simulink model "RampModelRunner"  (R2017b)
settings: Solver=FixedStepDiscrete  StartTime=0.0  StopTime=10  FixedStep=0.02  RelTol=1e-3
undefined symbols (not defined in the file): C_CieCurveGammaToPwmY, C_CieCurvePwmToGammaY
libraries: Ramp_Library_R2017b x8, simulink x4
settings Model: DataDictionary=Ramp_Lib.sldd  PauseTimes=4  Creator=mchawa  LastModifiedBy=mchawa

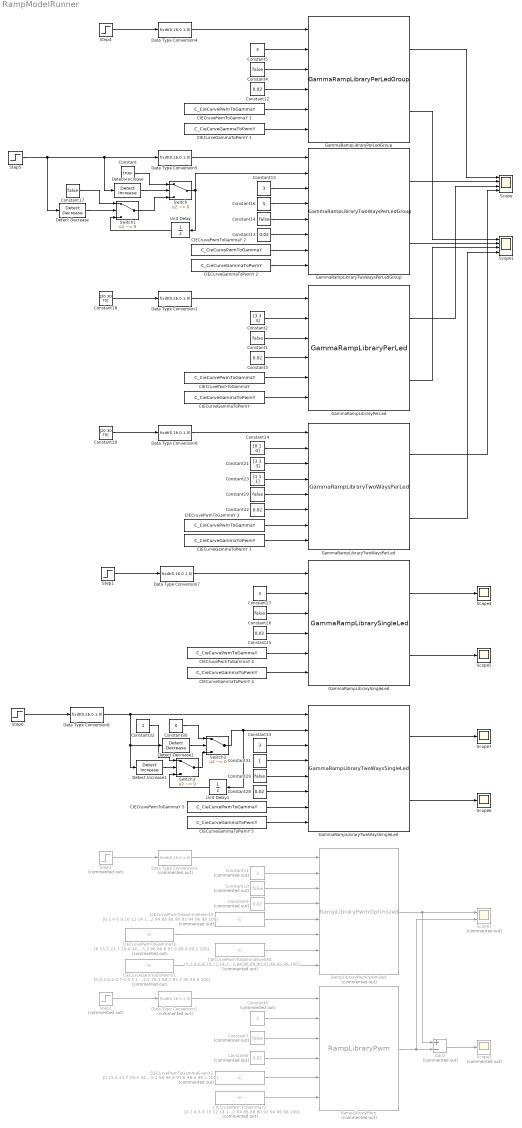
== system RampModelRunner ==
  Add1 : Sum  Commented=on  Inputs=+-  OutDataTypeStr=double
  CIECruvePwmToGammaY {,1..5} (6 alike) : Constant  Value=C_CieCurvePwmToGammaY
  CIECruvePwmToGammaY1 : Constant  Commented=on  Value="[0\t2\t4\t6\t8\t10\t12\t14\t16\t18\t20\t22\t24\t26\t28\t30\t32\t34\t36\t38\t40\t42\t44\t46\t48\t50\t52\t54\t56\t58\t60\t62\t64\t66\t68\t70\t72\t74\t76\t78\t80\t82\t84\t86\t88\t90\t92\t94\t96\t98\t100]"  OutDataTypeStr=fixdt(0,16,0.1,0)
  CIECruvePwmToGammaY3 : Constant  Commented=on  Value=[0 15.5 23.7 29.4 34 37.8 41.2 44.2 47 49.5 51.8 54 56.1 58 59.9 61.7 63.3 65 66.5 68 69.5 70.9 72.2 73.5 74.8 76.1 77.3 78.5 79.6 80.7 81.8 82.9 84 85 86 87 88 88.9 89.9 90.8 91.7 92.6 93.5 94.3 95.2 96 96.8 97.6 98.4 99.2 100]  OutDataTypeStr=fixdt(0,16,0.1,0)
  CIECurveGammaToPwmY {,1..5} (6 alike) : Constant  Value=C_CieCurveGammaToPwmY
  CIECurveGammaToPwmY1 : Constant  Commented=on  Value=[0 0.2 0.4 0.7 0.9 1.1 1.4 1.7 2.1 2.5 3 3.5 4.1 4.7 5.5 6.2 7.1 8 9 10.1 11.3 12.5 13.8 15.3 16.8 18.4 20.1 22 23.9 26 28.1 30.4 32.8 35.3 38 40.7 43.7 46.7 49.9 53.2 56.7 60.3 64.1 68 72.1 76.3 80.7 85.3 90 94.9 100]  OutDataTypeStr=fixdt(0,16,0.1,0)
  CIECurvePwmToGammaEvenX1 : Constant  Commented=on  Value=[0 15.5 23.7 29.4 34 37.8 41.2 44.2 47 49.5 51.8 54 56.1 58 59.9 61.7 63.3 65 66.5 68 69.5 70.9 72.2 73.5 74.8 76.1 77.3 78.5 79.6 80.7 81.8 82.9 84 85 86 87 88 88.9 89.9 90.8 91.7 92.6 93.5 94.3 95.2 96 96.8 97.6 98.4 99.2 100]  OutDataTypeStr=fixdt(0,16,0.1,0)
  CIECurvePwmToGammaEvenX3 : Constant  Commented=on  Value=[0 2 4 6 8 10 12 14 16 18 20 22 24 26 28 30 32 34 36 38 40 42 44 46 48 50 52 54 56 58 60 62 64 66 68 70 72 74 76 78 80 82 84 86 88 90 92 94 96 98 100]  OutDataTypeStr=uint8
  CIECurvePwmToGammaEvenX4 : Constant  Commented=on  Value=[0 2 4 6 8 10 12 14 16 18 20 22 24 26 28 30 32 34 36 38 40 42 44 46 48 50 52 54 56 58 60 62 64 66 68 70 72 74 76 78 80 82 84 86 88 90 92 94 96 98 100]  OutDataTypeStr=uint8
  Constant : Constant  Value=true  OutDataTypeStr=boolean
  Constant{1,4,14,19,26,29} (6 alike) : Constant  Value=false
  Constant10 : Constant  Commented=on  Value=false
  Constant11 : Constant  Commented=on  Value=3  OutDataTypeStr=fixdt(0,16,0.005,0)
  Constant{3,12..13,22,25,28} (6 alike) : Constant  Value=0.02  OutDataTypeStr=fixdt(0,16,0.005,0)
  Constant{5,15,27,33} (4 alike) : Constant  Value=3  OutDataTypeStr=fixdt(0,16,0.005,0)
  Constant16 : Constant  Value=5  OutDataTypeStr=fixdt(0,16,0.005,0)
  Constant17 : Constant  Value=false  OutDataTypeStr=boolean
  Constant18 : Constant  Value=[20 30 70]
  Constant2 : Constant  Value=[3 3 3]  OutDataTypeStr=fixdt(0,16,0.005,0)
  Constant20 : Constant  Value=[20 30 70]
  Constant21 : Constant  Value=[3 3 3]  OutDataTypeStr=fixdt(0,16,0.005,0)
  Constant23 : Constant  Value=[1 1 1]  OutDataTypeStr=fixdt(0,16,0.005,0)
  Constant24 : Constant  Value=[0 1 0]  OutDataTypeStr=boolean
  Constant30 : Constant  Value=0  OutDataTypeStr=fixdt(0,16,0.005,0)
  Constant31 : Constant  OutDataTypeStr=fixdt(0,16,0.005,0)
  Constant32 : Constant  OutDataTypeStr=fixdt(0,16,0.005,0)
  Constant6 : Constant  Commented=on  Value=0.02  OutDataTypeStr=fixdt(0,16,0.005,0)
  Constant7 : Constant  Commented=on  Value=false
  Constant8 : Constant  Commented=on  Value=3  OutDataTypeStr=fixdt(0,16,0.005,0)
  Constant9 : Constant  Commented=on  Value=0.02  OutDataTypeStr=fixdt(0,16,0.005,0)
  Data Type Conversion{1,4..8} (6 alike) : DataTypeConversion  OutDataTypeStr=fixdt(0,16,0.1,0)
  Data Type Conversion2 : DataTypeConversion  Commented=on  OutDataTypeStr=fixdt(0,16,0.1,0)
  Data Type Conversion3 : DataTypeConversion  Commented=on  OutDataTypeStr=fixdt(0,16,0.1,0)
  Detect Decrease : simulink/Logic and Bit Operations/Detect Decrease  vinit=0.0  OutDataTypeStr=boolean
  Detect Decrease1 : simulink/Logic and Bit Operations/Detect Decrease  vinit=0.0  OutDataTypeStr=boolean
  Detect Increase : simulink/Logic and Bit Operations/Detect Increase  vinit=0.0  OutDataTypeStr=boolean
  Detect Increase1 : simulink/Logic and Bit Operations/Detect Increase  vinit=0.0  OutDataTypeStr=boolean
  GammaRampLibraryPerLed : Ramp_Library_R2017b/GammaRampLibraryPerLed  Description=|
      | This library performs ramp function taking CIE curves which are evenly distributed.
      | It performs the ramp linearly on the Gamma Curve.
  GammaRampLibraryPerLedGroup : Ramp_Library_R2017b/GammaRampLibraryPerLedGroup  Description=|
      | This library performs ramp function taking CIE curves which are evenly distributed.
      | It performs the ramp linearly on the Gamma Curve.
  GammaRampLibrarySingleLed : Ramp_Library_R2017b/GammaRampLibrarySingleLed  Description=|
      | This library performs ramp function taking CIE curves which are evenly distributed.
      | It performs the ramp linearly on the Gamma Curve.
  GammaRampLibraryTwoWaysPerLed : Ramp_Library_R2017b/GammaRampLibraryTwoWaysPerLed  Description=|
      | This library performs ramp function taking CIE curves which are evenly distributed.
      | It performs the ramp linearly on the Gamma Curve.
  GammaRampLibraryTwoWaysPerLedGroup : Ramp_Library_R2017b/GammaRampLibraryTwoWaysPerLedGroup  Description=|
      | This library performs ramp function taking CIE curves which are evenly distributed.
      | It performs the ramp linearly on the Gamma Curve.
  GammaRampLibraryTwoWaysSingleLed : Ramp_Library_R2017b/GammaRampLibraryTwoWaysSingleLed  Description=|
      | This library performs ramp function taking CIE curves which are evenly distributed.
      | It performs the ramp linearly on the Gamma Curve.
  RampLibraryPwm : Ramp_Library_R2017b/RampLibraryPwm  Commented=on
  RampLibraryPwmOptimized : Ramp_Library_R2017b/RampLibraryPwmOptimized  Commented=on
  Scope : Scope  NumInputPorts=4
  Scope1 : Scope  NumInputPorts=4
  Scope2 : Scope  Commented=on
  Scope3 : Scope  Commented=on  NumInputPorts=2
  Scope{4..7} (4 alike) : Scope
  Step1 : Step  Time=4  Before=50  After=0  SampleTime=0.02
  Step2 : Step  Commented=on  Time=4  Before=50  After=0  SampleTime=0.02
  Step3 : Step  Commented=on  Time=4  Before=50  After=0  SampleTime=0.02
  Step4 : Step  Time=4  Before=50  After=0  SampleTime=0.02
  Step5 : Step  Time=4  Before=50  After=0  SampleTime=0.02
  Step6 : Step  Time=4  Before=100  After=0  SampleTime=0.02
  Switch{,1..3} (4 alike) : Switch  Criteria=u2 ~= 0
  Unit Delay : UnitDelay  SampleTime=-1
  Unit Delay1 : UnitDelay  SampleTime=-1
  wires:
  Data Type Conversion2/1 -> RampLibraryPwm/1
  CIECruvePwmToGammaY1/1 -> RampLibraryPwm/6
  Constant6/1 -> RampLibraryPwm/4
  Constant8/1 -> RampLibraryPwm/2
  Constant7/1 -> RampLibraryPwm/3
  Step2/1 -> Data Type Conversion2/1
  CIECurvePwmToGammaEvenX1/1 -> RampLibraryPwm/5
  RampLibraryPwm/1 -> Add1/2, Scope3/2
  Step3/1 -> Data Type Conversion3/1
  Data Type Conversion3/1 -> RampLibraryPwmOptimized/1
  Constant11/1 -> RampLibraryPwmOptimized/2
  Constant10/1 -> RampLibraryPwmOptimized/3
  Constant9/1 -> RampLibraryPwmOptimized/4
  CIECurvePwmToGammaEvenX3/1 -> RampLibraryPwmOptimized/5
  CIECurvePwmToGammaEvenX4/1 -> RampLibraryPwmOptimized/7
  CIECruvePwmToGammaY3/1 -> RampLibraryPwmOptimized/6
  CIECurveGammaToPwmY1/1 -> RampLibraryPwmOptimized/8
  RampLibraryPwmOptimized/1 -> Add1/1, Scope3/1
  Add1/1 -> Scope2/1
  Data Type Conversion1/1 -> GammaRampLibraryPerLed/1
  Constant1/1 -> GammaRampLibraryPerLed/3
  Constant3/1 -> GammaRampLibraryPerLed/4
  Constant2/1 -> GammaRampLibraryPerLed/2
  Constant18/1 -> Data Type Conversion1/1
  "CIECruvePwmToGammaY "/1 -> GammaRampLibraryPerLed/5
  "CIECurveGammaToPwmY "/1 -> GammaRampLibraryPerLed/6
  Constant4/1 -> GammaRampLibraryPerLedGroup/3
  CIECruvePwmToGammaY 1/1 -> GammaRampLibraryPerLedGroup/5
  Data Type Conversion4/1 -> GammaRampLibraryPerLedGroup/1
  Step4/1 -> Data Type Conversion4/1
  Constant5/1 -> GammaRampLibraryPerLedGroup/2
  Constant12/1 -> GammaRampLibraryPerLedGroup/4
  CIECurveGammaToPwmY 1/1 -> GammaRampLibraryPerLedGroup/6
  Step5/1 -> Detect Decrease/1, Detect Increase/1, Data Type Conversion5/1
  Data Type Conversion5/1 -> GammaRampLibraryTwoWaysPerLedGroup/1
  Constant15/1 -> GammaRampLibraryTwoWaysPerLedGroup/3
  CIECurveGammaToPwmY 2/1 -> GammaRampLibraryTwoWaysPerLedGroup/8
  CIECruvePwmToGammaY 2/1 -> GammaRampLibraryTwoWaysPerLedGroup/7
  Constant13/1 -> GammaRampLibraryTwoWaysPerLedGroup/6
  Constant14/1 -> GammaRampLibraryTwoWaysPerLedGroup/5
  Constant16/1 -> GammaRampLibraryTwoWaysPerLedGroup/4
  Switch/1 -> GammaRampLibraryTwoWaysPerLedGroup/2, Unit Delay/1
  Detect Increase/1 -> Switch/2
  Constant/1 -> Switch/1
  Switch1/1 -> Switch/3
  Detect Decrease/1 -> Switch1/2
  Constant17/1 -> Switch1/1
  Unit Delay/1 -> Switch1/3
  GammaRampLibraryTwoWaysPerLedGroup/1 -> Scope/2
  GammaRampLibraryTwoWaysPerLedGroup/2 -> Scope1/2
  GammaRampLibraryPerLedGroup/1 -> Scope/1
  GammaRampLibraryPerLedGroup/2 -> Scope1/1
  GammaRampLibraryPerLed/1 -> Scope/3
  GammaRampLibraryPerLed/2 -> Scope1/3
  Data Type Conversion6/1 -> GammaRampLibraryTwoWaysPerLed/1
  Constant20/1 -> Data Type Conversion6/1
  CIECurveGammaToPwmY 3/1 -> GammaRampLibraryTwoWaysPerLed/8
  CIECruvePwmToGammaY 3/1 -> GammaRampLibraryTwoWaysPerLed/7
  Constant22/1 -> GammaRampLibraryTwoWaysPerLed/6
  Constant19/1 -> GammaRampLibraryTwoWaysPerLed/5
  Constant21/1 -> GammaRampLibraryTwoWaysPerLed/3
  Constant23/1 -> GammaRampLibraryTwoWaysPerLed/4
  Constant24/1 -> GammaRampLibraryTwoWaysPerLed/2
  GammaRampLibraryTwoWaysPerLed/2 -> Scope1/4
  GammaRampLibraryTwoWaysPerLed/1 -> Scope/4
  Step1/1 -> Data Type Conversion7/1
  Data Type Conversion7/1 -> GammaRampLibrarySingleLed/1
  Constant27/1 -> GammaRampLibrarySingleLed/2
  Constant26/1 -> GammaRampLibrarySingleLed/3
  Constant25/1 -> GammaRampLibrarySingleLed/4
  CIECruvePwmToGammaY 4/1 -> GammaRampLibrarySingleLed/5
  CIECurveGammaToPwmY 4/1 -> GammaRampLibrarySingleLed/6
  GammaRampLibrarySingleLed/1 -> Scope4/1
  GammaRampLibrarySingleLed/2 -> Scope5/1
  Data Type Conversion8/1 -> Detect Increase1/1, Detect Decrease1/1, GammaRampLibraryTwoWaysSingleLed/1
  CIECurveGammaToPwmY 5/1 -> GammaRampLibraryTwoWaysSingleLed/8
  Step6/1 -> Data Type Conversion8/1
  CIECruvePwmToGammaY 5/1 -> GammaRampLibraryTwoWaysSingleLed/7
  Constant28/1 -> GammaRampLibraryTwoWaysSingleLed/6
  Constant29/1 -> GammaRampLibraryTwoWaysSingleLed/5
  Detect Decrease1/1 -> Switch2/2
  Constant30/1 -> Switch2/1
  Detect Increase1/1 -> Switch3/2
  Switch3/1 -> Switch2/3
  Constant32/1 -> Switch3/1
  Switch2/1 -> Unit Delay1/1, GammaRampLibraryTwoWaysSingleLed/2
  Constant31/1 -> GammaRampLibraryTwoWaysSingleLed/4
  Constant33/1 -> GammaRampLibraryTwoWaysSingleLed/3
  Unit Delay1/1 -> Switch3/3
  GammaRampLibraryTwoWaysSingleLed/1 -> Scope7/1
  GammaRampLibraryTwoWaysSingleLed/2 -> Scope6/1
